simulink model "multipleRateExample"  (R2023a)
settings: Solver=FixedStepAuto  StartTime=0.0  StopTime=inf  RelTol=1e-3
undefined symbols (not defined in the file): Payload
libraries: uavmavlinklib x8, simulink_extras x3, aerolibanimutils x1, instrumentlib x1
settings Model: Creator=Alireza  LastModifiedBy=Alireza

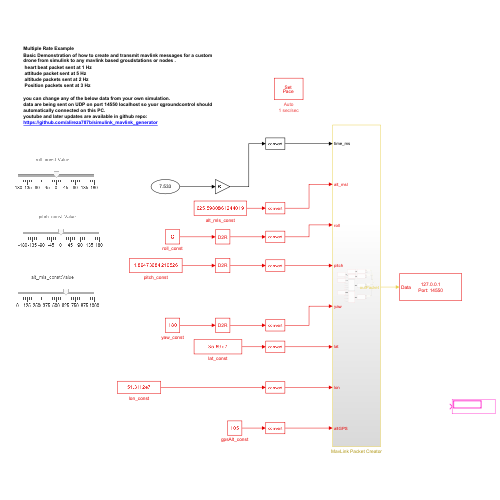
[thumbnail: Simulink's stored preview of the top-level diagram]
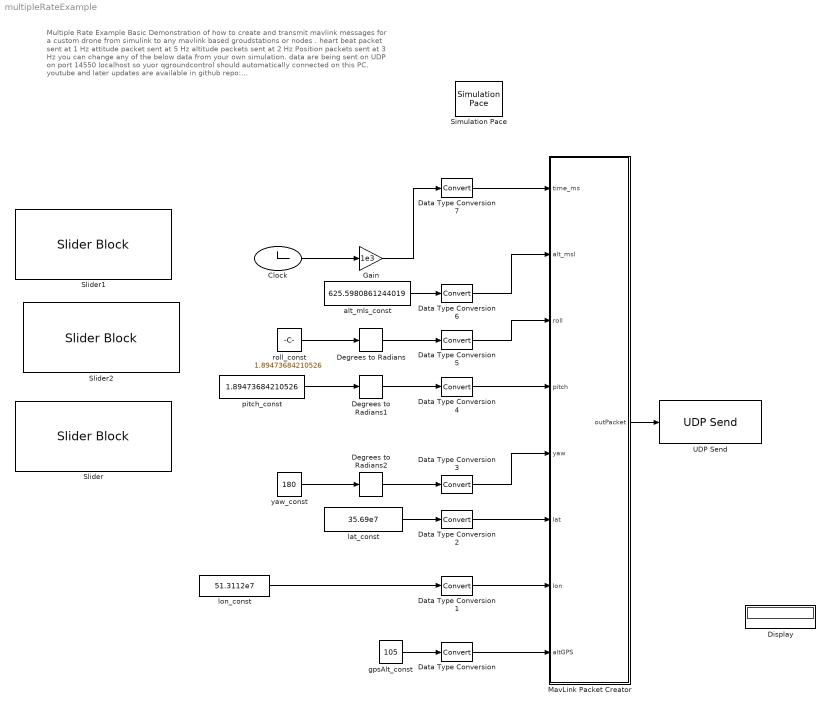
== system multipleRateExample ==
  note: Multiple Rate Example
      | Basic Demonstration of how to create and transmit mavlink messages for a custom drone from simulink to any mavlink based groudstations or nodes .
      | heart beat packet sent at 1 Hz
      | attitude packet sent at 5 Hz
      | altitude packets sent at 2 Hz
      | Position packets sent at 3 Hz
      |
      | you can change any of the below data from your own simulation.
      | data are being sent on UDP on port 14550 localhost so yuor qgroundcontrol should automatically connected on this PC.
      | youtube and later updates are available in github repo:
      | https://github.com/alireza787b/simulink_mavlink_generator
  Clock : Clock
      settings: Decimation=3
  Data Type Conversion{,1..7} (8 alike) : DataTypeConversion  SaturateOnIntegerOverflow=off  RndMeth=Floor
  Degrees to Radians : simulink_extras/Transformations/Degrees to Radians
  Degrees to Radians1 : simulink_extras/Transformations/Degrees to Radians
  Degrees to Radians2 : simulink_extras/Transformations/Degrees to Radians
  Display : Display
  Gain : Gain  Gain=1e3
  MavLink Packet Creator : Subsystem
  Simulation Pace : aerolibanimutils/Simulation Pace  SimulationPace=1  SleepMode=Auto  OutputPaceError=off  SampleTime=-1
  Slider : SliderBlock  ScaleMax=1000
  Slider1 : SliderBlock  ScaleMin=-180  ScaleMax=180
  Slider2 : SliderBlock  ScaleMin=-180  ScaleMax=180
  UDP Send : instrumentlib/UDP Send  Host=127.0.0.1  Port=14550  LocalAddress=127.0.0.1  LocalPort=-1  EnablePortSharing=off  OutputDatagramPacketSize=512  ByteOrder=big-endian  EnableBlockingMode=off  SimulateUsing=Interpreted execution
  alt_mls_const : Constant  Value=625.5980861244019  SampleTime=-1
  gpsAlt_const : Constant  Value=105  SampleTime=-1
  lat_const : Constant  Value=35.69e7  SampleTime=-1
  lon_const : Constant  Value=51.3112e7  SampleTime=-1
  pitch_const : Constant  Value=1.89473684210526  SampleTime=-1
  roll_const : Constant  Value=1.89473684210526  SampleTime=-1
  yaw_const : Constant  Value=180  SampleTime=-1
  wires:
  lat_const/1 -> Data Type Conversion2/1
  Clock/1 -> Gain/1
  Data Type Conversion4/1 -> MavLink Packet Creator/4(pitch)
  Data Type Conversion6/1 -> MavLink Packet Creator/2(alt_msl)
  roll_const/1 -> Degrees to Radians/1
  yaw_const/1 -> Degrees to Radians2/1
  Degrees to Radians1/1 -> Data Type Conversion4/1
  alt_mls_const/1 -> Data Type Conversion6/1
  pitch_const/1 -> Degrees to Radians1/1
  Gain/1 -> Data Type Conversion7/1
  Degrees to Radians/1 -> Data Type Conversion5/1
  Degrees to Radians2/1 -> Data Type Conversion3/1
  lon_const/1 -> Data Type Conversion1/1
  gpsAlt_const/1 -> Data Type Conversion/1
  MavLink Packet Creator/1(outPacket) -> UDP Send/1
  Data Type Conversion7/1 -> MavLink Packet Creator/1(time_ms)
  Data Type Conversion5/1 -> MavLink Packet Creator/3(roll)
  Data Type Conversion1/1 -> MavLink Packet Creator/7(lon)
  Data Type Conversion3/1 -> MavLink Packet Creator/5(yaw)
  Data Type Conversion/1 -> MavLink Packet Creator/8(altGPS)
  Data Type Conversion2/1 -> MavLink Packet Creator/6(lat)

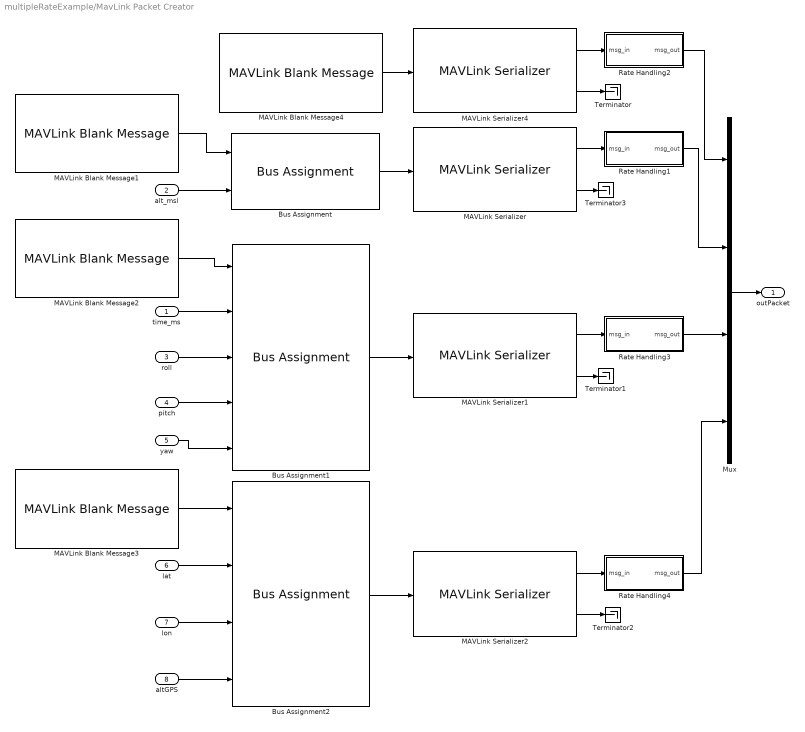
== system multipleRateExample/MavLink Packet Creator ==
  time_ms : Inport
  alt_msl : Inport  Port=2
  roll : Inport  Port=3
  pitch : Inport  Port=4
  yaw : Inport  Port=5
  lat : Inport  Port=6
  lon : Inport  Port=7
  altGPS : Inport  Port=8
  Bus Assignment : BusAssignment  AssignedSignals=Payload.altitude_amsl
  Bus Assignment1 : BusAssignment  AssignedSignals=Payload.time_boot_ms,Payload.roll,Payload.pitch,Payload.yaw
  Bus Assignment2 : BusAssignment  AssignedSignals=Payload.lat,Payload.lon,Payload.alt
  MAVLink Blank Message1 : uavmavlinklib/MAVLink Blank Message  dialectSource=Select from standard MAVLink dialects  dialect=common.xml  dialectCustom=common.xml  version=2  messageType=ALTITUDE  SystemID=2  ComponentID=1  SampleTime=-1
  MAVLink Blank Message2 : uavmavlinklib/MAVLink Blank Message  dialectSource=Select from standard MAVLink dialects  dialect=common.xml  dialectCustom=common.xml  version=2  messageType=ATTITUDE  SystemID=2  ComponentID=1  SampleTime=-1
  MAVLink Blank Message3 : uavmavlinklib/MAVLink Blank Message  dialectSource=Select from standard MAVLink dialects  dialect=common.xml  dialectCustom=common.xml  version=2  messageType=GLOBAL_POSITION_INT  SystemID=2  ComponentID=1  SampleTime=-1
  MAVLink Blank Message4 : uavmavlinklib/MAVLink Blank Message  dialectSource=Select from standard MAVLink dialects  dialect=common.xml  dialectCustom=common.xml  version=2  messageType=HEARTBEAT  SystemID=2  ComponentID=1  SampleTime=-1
  MAVLink Serializer : uavmavlinklib/MAVLink Serializer  dialectSource=Select from standard MAVLink dialects  dialect=common.xml  dialectCustom=common.xml  version=2  messageType=ALTITUDE
  MAVLink Serializer1 : uavmavlinklib/MAVLink Serializer  dialectSource=Select from standard MAVLink dialects  dialect=common.xml  dialectCustom=common.xml  version=2  messageType=ATTITUDE
  MAVLink Serializer2 : uavmavlinklib/MAVLink Serializer  dialectSource=Select from standard MAVLink dialects  dialect=common.xml  dialectCustom=common.xml  version=2  messageType=GLOBAL_POSITION_INT
  MAVLink Serializer4 : uavmavlinklib/MAVLink Serializer  dialectSource=Select from standard MAVLink dialects  dialect=common.xml  dialectCustom=common.xml  version=2  messageType=HEARTBEAT
  Mux : Mux
  Rate Handling1 : Subsystem  mask{Sample_Rate=2}
      mask prompts: Sample_Rate "Sample Rate"
  Rate Handling2 : Subsystem  mask{Sample_Rate=1}
      mask prompts: Sample_Rate "Sample Rate"
  Rate Handling3 : Subsystem  mask{Sample_Rate=5}
      mask prompts: Sample_Rate "Sample Rate"
  Rate Handling4 : Subsystem  mask{Sample_Rate=3}
      mask prompts: Sample_Rate "Sample Rate"
  Terminator{,1..3} (4 alike) : Terminator
  outPacket : Outport
  wires:
  MAVLink Blank Message1/1 -> Bus Assignment/1
  alt_msl/1 -> Bus Assignment/2
  Rate Handling4/1(msg_out) -> Mux/4
  MAVLink Blank Message3/1 -> Bus Assignment2/1
  time_ms/1 -> Bus Assignment1/2
  MAVLink Blank Message2/1 -> Bus Assignment1/1
  Bus Assignment/1 -> MAVLink Serializer/1
  roll/1 -> Bus Assignment1/3
  pitch/1 -> Bus Assignment1/4
  yaw/1 -> Bus Assignment1/5
  MAVLink Serializer1/1 -> Rate Handling3/1(msg_in)
  lat/1 -> Bus Assignment2/2
  Rate Handling3/1(msg_out) -> Mux/3
  lon/1 -> Bus Assignment2/3
  altGPS/1 -> Bus Assignment2/4
  MAVLink Blank Message4/1 -> MAVLink Serializer4/1
  Bus Assignment1/1 -> MAVLink Serializer1/1
  Bus Assignment2/1 -> MAVLink Serializer2/1
  MAVLink Serializer4/1 -> Rate Handling2/1(msg_in)
  MAVLink Serializer/1 -> Rate Handling1/1(msg_in)
  MAVLink Serializer2/1 -> Rate Handling4/1(msg_in)
  Rate Handling2/1(msg_out) -> Mux/1
  Rate Handling1/1(msg_out) -> Mux/2
  Mux/1 -> outPacket/1
  MAVLink Serializer4/2 -> Terminator/1
  MAVLink Serializer1/2 -> Terminator1/1
  MAVLink Serializer2/2 -> Terminator2/1
  MAVLink Serializer/2 -> Terminator3/1

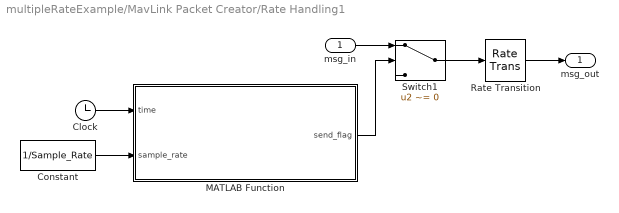
== system multipleRateExample/MavLink Packet Creator/Rate Handling1 ==
  msg_in : Inport
  Clock : Clock
      settings: Decimation=3
  Constant : Constant  Value=1/Sample_Rate  SampleTime=-1
  MATLAB Function : MATLAB Function  TreatAsAtomicUnit=on
  Rate Transition : RateTransition  Integrity=off  OutPortSampleTime=1/Sample_Rate
  Switch1 : Switch  Criteria=u2 ~= 0  Threshold=1/Sample_Rate  SaturateOnIntegerOverflow=off  InputSameDT=off
  msg_out : Outport
  wires:
  Rate Transition/1 -> msg_out/1
  MATLAB Function/1(send_flag) -> Switch1/2
  Constant/1 -> MATLAB Function/2(sample_rate)
  Switch1/1 -> Rate Transition/1
  Clock/1 -> MATLAB Function/1(time)
  msg_in/1 -> Switch1/1

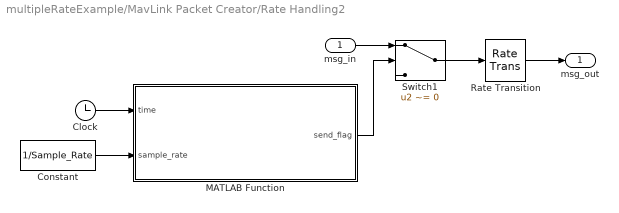
== system multipleRateExample/MavLink Packet Creator/Rate Handling2 ==
  msg_in : Inport
  Clock : Clock
      settings: Decimation=3
  Constant : Constant  Value=1/Sample_Rate  SampleTime=-1
  MATLAB Function : MATLAB Function  TreatAsAtomicUnit=on
  Rate Transition : RateTransition  Integrity=off  OutPortSampleTime=1/Sample_Rate
  Switch1 : Switch  Criteria=u2 ~= 0  Threshold=1/Sample_Rate  SaturateOnIntegerOverflow=off  InputSameDT=off
  msg_out : Outport
  wires:
  msg_in/1 -> Switch1/1
  Clock/1 -> MATLAB Function/1(time)
  Switch1/1 -> Rate Transition/1
  Constant/1 -> MATLAB Function/2(sample_rate)
  MATLAB Function/1(send_flag) -> Switch1/2
  Rate Transition/1 -> msg_out/1

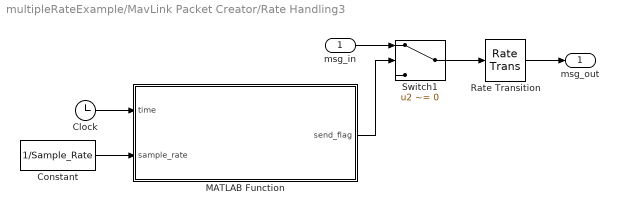
== system multipleRateExample/MavLink Packet Creator/Rate Handling3 ==
  msg_in : Inport
  Clock : Clock
      settings: Decimation=3
  Constant : Constant  Value=1/Sample_Rate  SampleTime=-1
  MATLAB Function : MATLAB Function  TreatAsAtomicUnit=on
  Rate Transition : RateTransition  Integrity=off  OutPortSampleTime=1/Sample_Rate
  Switch1 : Switch  Criteria=u2 ~= 0  Threshold=1/Sample_Rate  SaturateOnIntegerOverflow=off  InputSameDT=off
  msg_out : Outport
  wires:
  msg_in/1 -> Switch1/1
  Clock/1 -> MATLAB Function/1(time)
  Switch1/1 -> Rate Transition/1
  Constant/1 -> MATLAB Function/2(sample_rate)
  MATLAB Function/1(send_flag) -> Switch1/2
  Rate Transition/1 -> msg_out/1

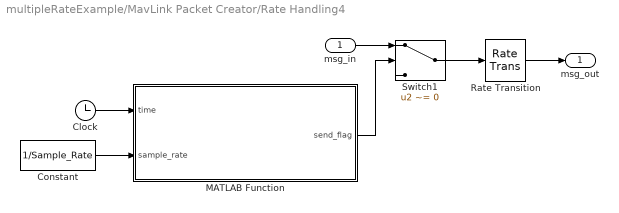
== system multipleRateExample/MavLink Packet Creator/Rate Handling4 ==
  msg_in : Inport
  Clock : Clock
      settings: Decimation=3
  Constant : Constant  Value=1/Sample_Rate  SampleTime=-1
  MATLAB Function : MATLAB Function  TreatAsAtomicUnit=on
  Rate Transition : RateTransition  Integrity=off  OutPortSampleTime=1/Sample_Rate
  Switch1 : Switch  Criteria=u2 ~= 0  Threshold=1/Sample_Rate  SaturateOnIntegerOverflow=off  InputSameDT=off
  msg_out : Outport
  wires:
  Rate Transition/1 -> msg_out/1
  MATLAB Function/1(send_flag) -> Switch1/2
  Constant/1 -> MATLAB Function/2(sample_rate)
  Switch1/1 -> Rate Transition/1
  Clock/1 -> MATLAB Function/1(time)
  msg_in/1 -> Switch1/1

== matlab function multipleRateExample/MavLink Packet Creator/Rate Handling1/MATLAB Function ==
  data: time input; send_flag output; sample_rate input
function send_flag = send_flag_creator(time,sample_rate)

persistent last_send;
if(isempty(last_send))
    last_send = 0;
end

if(time-last_send >= sample_rate)
    send_flag = true;
    last_send = time;
else
    send_flag = false;

end

== matlab function multipleRateExample/MavLink Packet Creator/Rate Handling3/MATLAB Function ==
  data: time input; send_flag output; sample_rate input
function send_flag = send_flag_creator(time,sample_rate)

persistent last_send;
if(isempty(last_send))
    last_send = 0;
end

if(time-last_send >= sample_rate)
    send_flag = true;
    last_send = time;
else
    send_flag = false;

end

== matlab function multipleRateExample/MavLink Packet Creator/Rate Handling4/MATLAB Function ==
  data: time input; send_flag output; sample_rate input
function send_flag = send_flag_creator(time,sample_rate)

persistent last_send;
if(isempty(last_send))
    last_send = 0;
end

if(time-last_send >= sample_rate)
    send_flag = true;
    last_send = time;
else
    send_flag = false;

end

== matlab function multipleRateExample/MavLink Packet Creator/Rate Handling2/MATLAB Function ==
  data: time input; send_flag output; sample_rate input
function send_flag = send_flag_creator(time,sample_rate)

persistent last_send;
if(isempty(last_send))
    last_send = 0;
end

if(time-last_send >= sample_rate)
    send_flag = true;
    last_send = time;
else
    send_flag = false;

end
